simulink model "LCL_Test"  (R2019b)
settings: Solver=VariableStepAuto  StartTime=0.0  StopTime=10  MaxStep=1e-6  RelTol=1e-3
values from neighbouring files (symbols this model uses):
  C_dhs = 300e-6    (= 0.0003)    [PHIL_dummy_motor.m]
  L_dhs = (720e-6)/2    (= 0.00036)    [PHIL_dummy_motor.m]
  L_drom = L    [PHIL_dummy_motor.m]
settings Model: Creator=kissd  LastModifiedBy=kissd

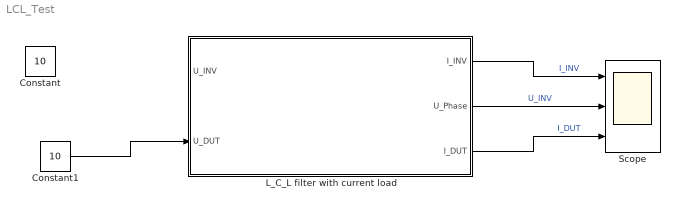
== system LCL_Test ==
  Constant : Constant  Value=10
  Constant1 : Constant  Value=10
  L_C_L filter with current load : Subsystem
  Scope : Scope  NumInputPorts=3
  wires:
  L_C_L filter with current load/2(U_Phase) -> Scope/2  "U_INV"
  L_C_L filter with current load/1(I_INV) -> Scope/1  "I_INV"
  L_C_L filter with current load/3(I_DUT) -> Scope/3  "I_DUT"
  ? -> L_C_L filter with current load/1(U_INV)
  Constant1/1 -> L_C_L filter with current load/2(U_DUT)

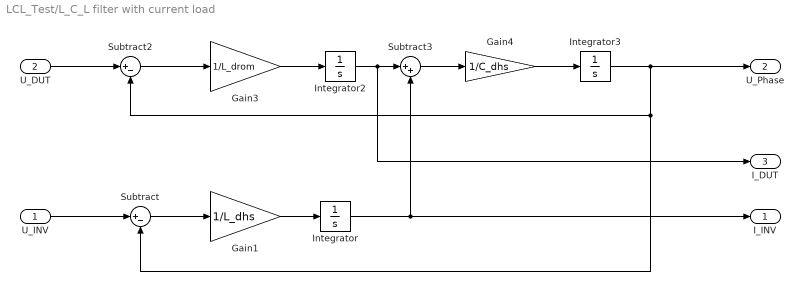
== system LCL_Test/L_C_L filter with current load ==
  U_INV : Inport
  U_DUT : Inport  Port=2
  Gain1 : Gain  Gain=1/L_dhs
  Gain3 : Gain  Gain=1/L_drom
  Gain4 : Gain  Gain=1/C_dhs
  Integrator : Integrator
  Integrator2 : Integrator
  Integrator3 : Integrator
  Subtract : Sum  Inputs=|+-
  Subtract2 : Sum  Inputs=|+-
  Subtract3 : Sum  Inputs=|++
  I_INV : Outport
  U_Phase : Outport  Port=2
  I_DUT : Outport  Port=3
  wires:
  Subtract/1 -> Gain1/1
  Gain1/1 -> Integrator/1
  Integrator/1 -> Subtract3/2, I_INV/1
  U_INV/1 -> Subtract/1
  U_DUT/1 -> Subtract2/1
  Subtract2/1 -> Gain3/1
  Gain3/1 -> Integrator2/1
  Integrator2/1 -> I_DUT/1, Subtract3/1
  Subtract3/1 -> Gain4/1
  Gain4/1 -> Integrator3/1
  Integrator3/1 -> Subtract2/2, Subtract/2, U_Phase/1
